simulink library "sysgenMatrixInversionLib"  (Simulink 7.5)
settings: Solver=ode45  StartTime=0.0  StopTime=10.0  RelTol=1e-3
libraries: xbsIndex_r4 x51
settings Model: Creator=arvinds  LastModifiedBy=arvinds

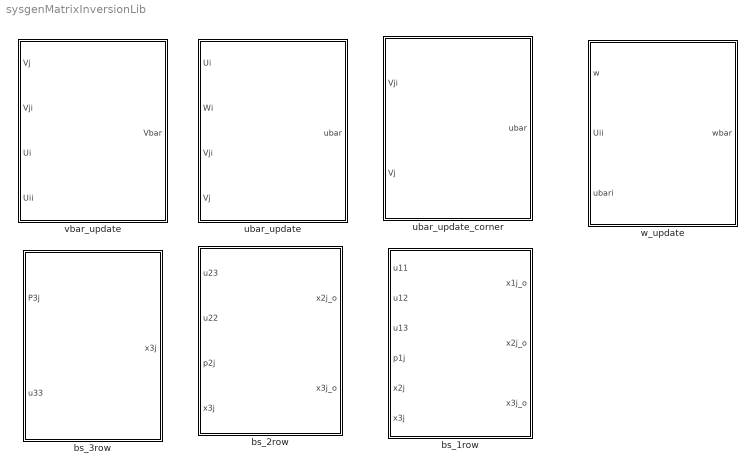
== system sysgenMatrixInversionLib ==
  bs_1row : Subsystem  mask{Latency=4}
      mask prompts: Latency "Primitive latency"
  bs_2row : Subsystem  mask{Latency=4}
      mask prompts: Latency "Primitive latency"
  bs_3row : Subsystem  mask{Latency=4}
      mask prompts: Latency "Primitive latency"
  ubar_update : Subsystem  mask{Latency=4}
      mask prompts: Latency "Primitive Latency"
  ubar_update_corner : Subsystem  mask{Latency=4}
      mask prompts: Latency "Primitive Latency"
  vbar_update : Subsystem  mask{Latency=4}
      mask prompts: Latency "Primitive Latency"
  w_update : Subsystem  mask{Latency=4}
      mask prompts: Latency "Primitive Latency"

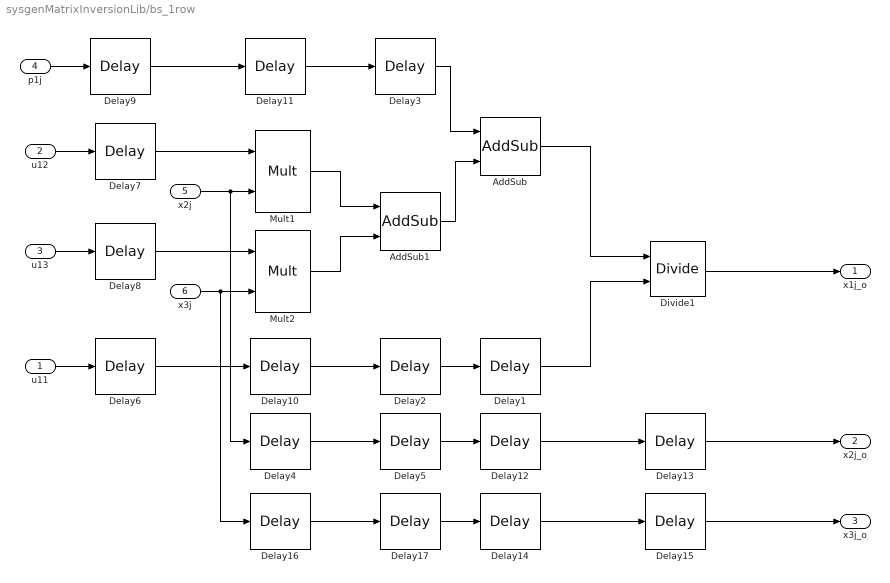
== system sysgenMatrixInversionLib/bs_1row ==
  u11 : Inport
  u12 : Inport  Port=2
  u13 : Inport  Port=3
  p1j : Inport  Port=4
  x2j : Inport  Port=5
  x3j : Inport  Port=6
  AddSub : xbsIndex_r4/AddSub  mode=Subtraction  use_carryin=off  use_carryout=off  en=off  latency=Latency  precision=Full  arith_type=Unsigned  n_bits=16  bin_pt=14  quantization=Truncate  overflow=Wrap  dbl_ovrd=off  use_behavioral_HDL=off  hw_selection=Fabric  pipelined=off  block_type=addsub
  AddSub1 : xbsIndex_r4/AddSub  mode=Addition  use_carryin=off  use_carryout=off  en=off  latency=Latency  precision=Full  arith_type=Unsigned  n_bits=16  bin_pt=14  quantization=Truncate  overflow=Wrap  dbl_ovrd=off  use_behavioral_HDL=off  hw_selection=Fabric  pipelined=off  block_type=addsub
  Delay{1..5,10..17} (13 alike) : xbsIndex_r4/Delay  rst=off  infoeditControl=Selection of Reset will increase slice count due to use of real FFs and instead of SRLs  en=off  latency=Latency  dbl_ovrd=off  reg_retiming=off  block_type=delay
  Delay{6..9} (4 alike) : xbsIndex_r4/Delay  rst=off  infoeditControl=Selection of Reset will increase slice count due to use of real FFs and instead of SRLs  en=off  latency=4*Latency  dbl_ovrd=off  reg_retiming=off  block_type=delay
  Divide1 : xbsIndex_r4/Divide  flow_control=NonBlocking  axi_optimize_goal=Resources  algorithm_type=High_Radix  infoedit1=Specify output fraction-width for Fixed-point division.  fractional_width=16  latency=Latency  rate=1  has_a_tlast=off  has_a_tuser=off  has_b_tlast=off  has_b_tuser=off  en=off  has_result_tready=off  result_tlast_behv=Pass_A_TLAST  has_underflow=off  has_overflow=off  has_invalid_op=off  has_divide_by_zero=off  fpo_op_type=mergeddivide  block_type=divide
      settings: infoedit=Blocking: Wait for data on all inputs, allow back-pressure.<br>NonBlocking: operate every cycle in which all inputs are valid, no back-pressure.
  Mult1 : xbsIndex_r4/Mult  precision=Full  arith_type="Signed  (2's comp)"  n_bits=16  bin_pt=14  quantization=Truncate  overflow=Wrap  en=off  latency=Latency  dbl_ovrd=off  use_behavioral_HDL=off  opt=Speed  use_embedded=on  optimum_pipeline=off  pipeline=on  use_rpm=on  placement_style=Triangular  block_type=mult
  Mult2 : xbsIndex_r4/Mult  precision=Full  arith_type="Signed  (2's comp)"  n_bits=16  bin_pt=14  quantization=Truncate  overflow=Wrap  en=off  latency=Latency  dbl_ovrd=off  use_behavioral_HDL=off  opt=Speed  use_embedded=on  optimum_pipeline=off  pipeline=on  use_rpm=on  placement_style=Triangular  block_type=mult
  x1j_o : Outport
  x2j_o : Outport  Port=2
  x3j_o : Outport  Port=3
  wires:
  u11/1 -> Delay6/1
  u12/1 -> Delay7/1
  u13/1 -> Delay8/1
  p1j/1 -> Delay9/1
  Delay7/1 -> Mult1/1
  x2j/1 -> Mult1/2, Delay4/1
  Delay8/1 -> Mult2/1
  x3j/1 -> Mult2/2, Delay16/1
  Delay6/1 -> Delay10/1
  Delay9/1 -> Delay11/1
  Mult1/1 -> AddSub1/1
  Mult2/1 -> AddSub1/2
  Delay10/1 -> Delay2/1
  Delay11/1 -> Delay3/1
  Delay3/1 -> AddSub/1
  AddSub1/1 -> AddSub/2
  AddSub/1 -> Divide1/1
  Delay2/1 -> Delay1/1
  Delay1/1 -> Divide1/2
  Divide1/1 -> x1j_o/1
  Delay4/1 -> Delay5/1
  Delay5/1 -> Delay12/1
  Delay12/1 -> Delay13/1
  Delay13/1 -> x2j_o/1
  Delay16/1 -> Delay17/1
  Delay17/1 -> Delay14/1
  Delay14/1 -> Delay15/1
  Delay15/1 -> x3j_o/1

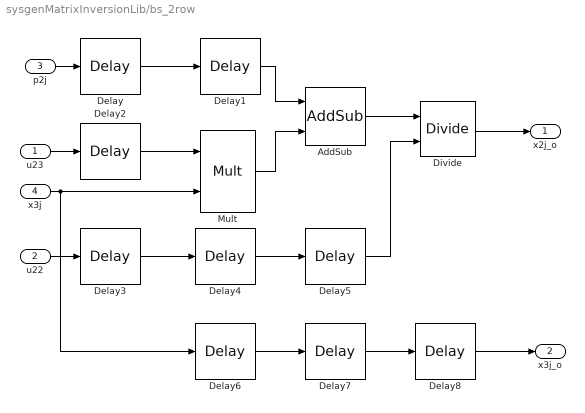
== system sysgenMatrixInversionLib/bs_2row ==
  u23 : Inport
  u22 : Inport  Port=2
  p2j : Inport  Port=3
  x3j : Inport  Port=4
  AddSub : xbsIndex_r4/AddSub  mode=Subtraction  use_carryin=off  use_carryout=off  en=off  latency=Latency  precision=Full  arith_type=Unsigned  n_bits=16  bin_pt=14  quantization=Truncate  overflow=Wrap  dbl_ovrd=off  use_behavioral_HDL=off  hw_selection=Fabric  pipelined=off  block_type=addsub
  Delay{,1..8} (9 alike) : xbsIndex_r4/Delay  rst=off  infoeditControl=Selection of Reset will increase slice count due to use of real FFs and instead of SRLs  en=off  latency=Latency  dbl_ovrd=off  reg_retiming=off  block_type=delay
  Divide : xbsIndex_r4/Divide  flow_control=NonBlocking  axi_optimize_goal=Resources  algorithm_type=High_Radix  infoedit1=Specify output fraction-width for Fixed-point division.  fractional_width=16  latency=Latency  rate=1  has_a_tlast=off  has_a_tuser=off  has_b_tlast=off  has_b_tuser=off  en=off  has_result_tready=off  result_tlast_behv=Pass_A_TLAST  has_underflow=off  has_overflow=off  has_invalid_op=off  has_divide_by_zero=off  fpo_op_type=mergeddivide  block_type=divide
      settings: infoedit=Blocking: Wait for data on all inputs, allow back-pressure.<br>NonBlocking: operate every cycle in which all inputs are valid, no back-pressure.
  Mult : xbsIndex_r4/Mult  precision=Full  arith_type="Signed  (2's comp)"  n_bits=16  bin_pt=14  quantization=Truncate  overflow=Wrap  en=off  latency=Latency  dbl_ovrd=off  use_behavioral_HDL=off  opt=Speed  use_embedded=on  optimum_pipeline=off  pipeline=on  use_rpm=on  placement_style=Triangular  block_type=mult
  x2j_o : Outport
  x3j_o : Outport  Port=2
  wires:
  Divide/1 -> x2j_o/1
  p2j/1 -> Delay/1
  Delay/1 -> Delay1/1
  u23/1 -> Delay2/1
  x3j/1 -> Mult/2, Delay6/1
  Delay2/1 -> Mult/1
  Delay1/1 -> AddSub/1
  Mult/1 -> AddSub/2
  AddSub/1 -> Divide/1
  u22/1 -> Delay3/1
  Delay3/1 -> Delay4/1
  Delay4/1 -> Delay5/1
  Delay5/1 -> Divide/2
  Delay8/1 -> x3j_o/1
  Delay6/1 -> Delay7/1
  Delay7/1 -> Delay8/1

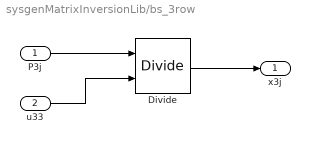
== system sysgenMatrixInversionLib/bs_3row ==
  P3j : Inport
  u33 : Inport  Port=2
  Divide : xbsIndex_r4/Divide  flow_control=NonBlocking  axi_optimize_goal=Resources  algorithm_type=High_Radix  infoedit1=Specify output fraction-width for Fixed-point division.  fractional_width=16  latency=Latency  rate=1  has_a_tlast=off  has_a_tuser=off  has_b_tlast=off  has_b_tuser=off  en=off  has_result_tready=off  result_tlast_behv=Pass_A_TLAST  has_underflow=off  has_overflow=off  has_invalid_op=off  has_divide_by_zero=off  fpo_op_type=mergeddivide  block_type=divide
      settings: infoedit=Blocking: Wait for data on all inputs, allow back-pressure.<br>NonBlocking: operate every cycle in which all inputs are valid, no back-pressure.
  x3j : Outport
  wires:
  P3j/1 -> Divide/1
  u33/1 -> Divide/2
  Divide/1 -> x3j/1

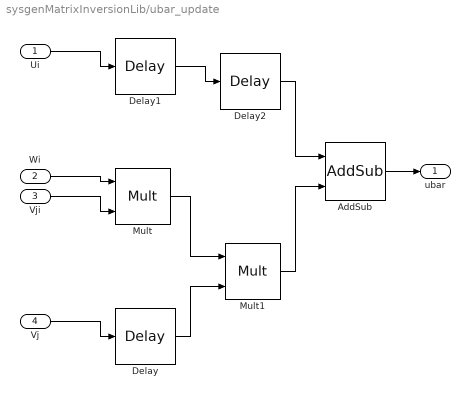
== system sysgenMatrixInversionLib/ubar_update ==
  Ui : Inport
  Wi : Inport  Port=2
  Vji : Inport  Port=3
  Vj : Inport  Port=4
  AddSub : xbsIndex_r4/AddSub  mode=Addition  use_carryin=off  use_carryout=off  en=off  latency=Latency  precision=Full  arith_type=Unsigned  n_bits=16  bin_pt=14  quantization=Truncate  overflow=Wrap  dbl_ovrd=off  use_behavioral_HDL=off  hw_selection=Fabric  pipelined=off  block_type=addsub
  Delay : xbsIndex_r4/Delay  rst=off  infoeditControl=Selection of Reset will increase slice count due to use of real FFs and instead of SRLs  en=off  latency=Latency  dbl_ovrd=off  reg_retiming=off  block_type=delay
  Delay1 : xbsIndex_r4/Delay  rst=off  infoeditControl=Selection of Reset will increase slice count due to use of real FFs and instead of SRLs  en=off  latency=Latency  dbl_ovrd=off  reg_retiming=off  block_type=delay
  Delay2 : xbsIndex_r4/Delay  rst=off  infoeditControl=Selection of Reset will increase slice count due to use of real FFs and instead of SRLs  en=off  latency=Latency  dbl_ovrd=off  reg_retiming=off  block_type=delay
  Mult : xbsIndex_r4/Mult  precision=Full  arith_type="Signed  (2's comp)"  n_bits=16  bin_pt=14  quantization=Truncate  overflow=Wrap  en=off  latency=Latency  dbl_ovrd=off  use_behavioral_HDL=off  opt=Speed  use_embedded=on  optimum_pipeline=off  pipeline=on  use_rpm=on  placement_style=Triangular  block_type=mult
  Mult1 : xbsIndex_r4/Mult  precision=Full  arith_type="Signed  (2's comp)"  n_bits=16  bin_pt=14  quantization=Truncate  overflow=Wrap  en=off  latency=Latency  dbl_ovrd=off  use_behavioral_HDL=off  opt=Speed  use_embedded=on  optimum_pipeline=off  pipeline=on  use_rpm=on  placement_style=Triangular  block_type=mult
  ubar : Outport
  wires:
  Wi/1 -> Mult/1
  Vji/1 -> Mult/2
  Vj/1 -> Delay/1
  Delay/1 -> Mult1/2
  Mult/1 -> Mult1/1
  Ui/1 -> Delay1/1
  Delay1/1 -> Delay2/1
  AddSub/1 -> ubar/1
  Delay2/1 -> AddSub/1
  Mult1/1 -> AddSub/2

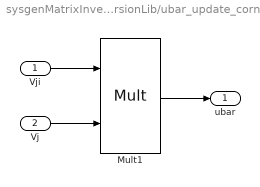
== system sysgenMatrixInversionLib/ubar_update_corner ==
  Vji : Inport
  Vj : Inport  Port=2
  Mult1 : xbsIndex_r4/Mult  precision=Full  arith_type="Signed  (2's comp)"  n_bits=16  bin_pt=14  quantization=Truncate  overflow=Wrap  en=off  latency=Latency  dbl_ovrd=off  use_behavioral_HDL=off  opt=Speed  use_embedded=on  optimum_pipeline=off  pipeline=on  use_rpm=on  placement_style=Triangular  block_type=mult
  ubar : Outport
  wires:
  Mult1/1 -> ubar/1
  Vj/1 -> Mult1/2
  Vji/1 -> Mult1/1

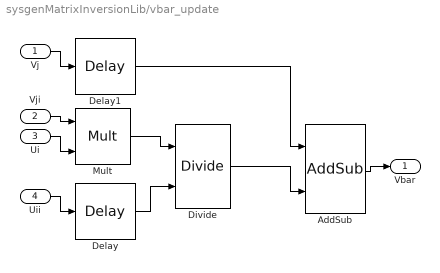
== system sysgenMatrixInversionLib/vbar_update ==
  Vj : Inport
  Vji : Inport  Port=2
  Ui : Inport  Port=3
  Uii : Inport  Port=4
  AddSub : xbsIndex_r4/AddSub  mode=Subtraction  use_carryin=off  use_carryout=off  en=off  latency=Latency  precision=Full  arith_type=Unsigned  n_bits=16  bin_pt=14  quantization=Truncate  overflow=Wrap  dbl_ovrd=off  use_behavioral_HDL=off  hw_selection=Fabric  pipelined=off  block_type=addsub
  Delay : xbsIndex_r4/Delay  rst=off  infoeditControl=Selection of Reset will increase slice count due to use of real FFs and instead of SRLs  en=off  latency=Latency  dbl_ovrd=off  reg_retiming=off  block_type=delay
  Delay1 : xbsIndex_r4/Delay  rst=off  infoeditControl=Selection of Reset will increase slice count due to use of real FFs and instead of SRLs  en=off  latency=2*Latency  dbl_ovrd=off  reg_retiming=off  block_type=delay
  Divide : xbsIndex_r4/Divide  flow_control=NonBlocking  axi_optimize_goal=Resources  algorithm_type=High_Radix  infoedit1=Specify output fraction-width for Fixed-point division.  fractional_width=16  latency=Latency  rate=1  has_a_tlast=off  has_a_tuser=off  has_b_tlast=off  has_b_tuser=off  en=off  has_result_tready=off  result_tlast_behv=Pass_A_TLAST  has_underflow=off  has_overflow=off  has_invalid_op=off  has_divide_by_zero=off  fpo_op_type=mergeddivide  block_type=divide
      settings: infoedit=Blocking: Wait for data on all inputs, allow back-pressure.<br>NonBlocking: operate every cycle in which all inputs are valid, no back-pressure.
  Mult : xbsIndex_r4/Mult  precision=Full  arith_type="Signed  (2's comp)"  n_bits=16  bin_pt=14  quantization=Truncate  overflow=Wrap  en=off  latency=Latency  dbl_ovrd=off  use_behavioral_HDL=off  opt=Speed  use_embedded=on  optimum_pipeline=off  pipeline=on  use_rpm=on  placement_style=Triangular  block_type=mult
  Vbar : Outport
  wires:
  Uii/1 -> Delay/1
  AddSub/1 -> Vbar/1
  Ui/1 -> Mult/2
  Vji/1 -> Mult/1
  Vj/1 -> Delay1/1
  Delay1/1 -> AddSub/1
  Delay/1 -> Divide/2
  Mult/1 -> Divide/1
  Divide/1 -> AddSub/2

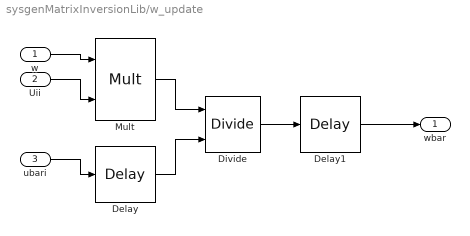
== system sysgenMatrixInversionLib/w_update ==
  w : Inport
  Uii : Inport  Port=2
  ubari : Inport  Port=3
  Delay : xbsIndex_r4/Delay  rst=off  infoeditControl=Selection of Reset will increase slice count due to use of real FFs and instead of SRLs  en=off  latency=Latency  dbl_ovrd=off  reg_retiming=off  block_type=delay
  Delay1 : xbsIndex_r4/Delay  rst=off  infoeditControl=Selection of Reset will increase slice count due to use of real FFs and instead of SRLs  en=off  latency=Latency  dbl_ovrd=off  reg_retiming=off  block_type=delay
  Divide : xbsIndex_r4/Divide  flow_control=NonBlocking  axi_optimize_goal=Resources  algorithm_type=Radix2  infoedit1=Specify output fraction-width for Fixed-point division.  fractional_width=16  latency=Latency  rate=1  has_a_tlast=off  has_a_tuser=off  has_b_tlast=off  has_b_tuser=off  en=off  has_result_tready=off  result_tlast_behv=Pass_A_TLAST  has_underflow=off  has_overflow=off  has_invalid_op=off  has_divide_by_zero=off  fpo_op_type=mergeddivide  block_type=divide
      settings: infoedit=Blocking: Wait for data on all inputs, allow back-pressure.<br>NonBlocking: operate every cycle in which all inputs are valid, no back-pressure.
  Mult : xbsIndex_r4/Mult  precision=Full  arith_type="Signed  (2's comp)"  n_bits=16  bin_pt=14  quantization=Truncate  overflow=Wrap  en=off  latency=Latency  dbl_ovrd=off  use_behavioral_HDL=off  opt=Speed  use_embedded=on  optimum_pipeline=off  pipeline=on  use_rpm=on  placement_style=Triangular  block_type=mult
  wbar : Outport
  wires:
  w/1 -> Mult/1
  Uii/1 -> Mult/2
  ubari/1 -> Delay/1
  Mult/1 -> Divide/1
  Delay/1 -> Divide/2
  Divide/1 -> Delay1/1
  Delay1/1 -> wbar/1
